simulink subsystem "DataSample"  (R2019b)
settings: Solver=VariableStepAuto  StartTime=0.0  StopTime=10.0  RelTol=1e-3
undefined symbols (not defined in the file or in its folder): __PRM__SERIALIZED__DATA__, SubsystemReferenceBlock
settings Model: Creator=VM  LastModifiedBy=VM

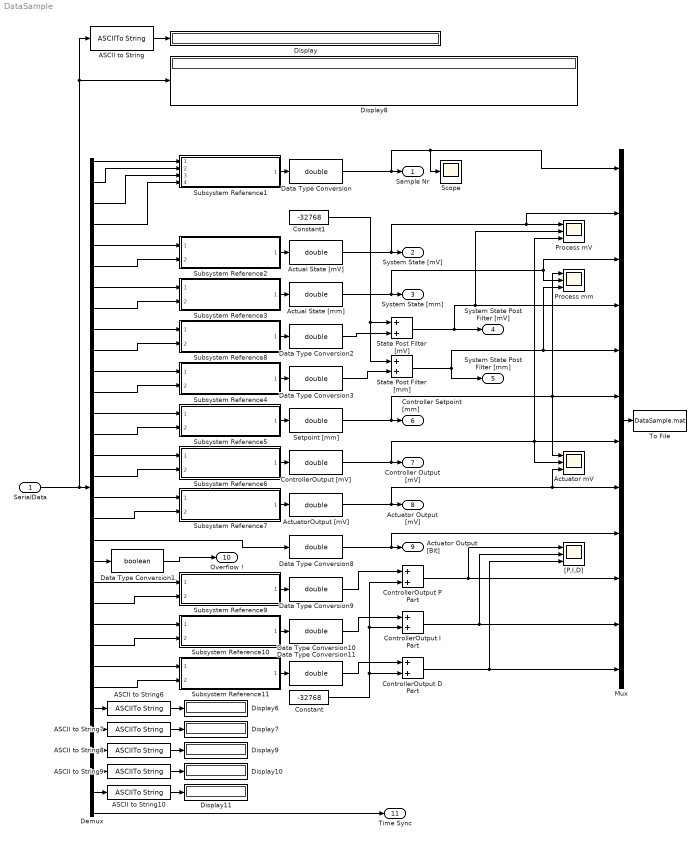
== system DataSample ==
  SerialData : Inport
  " Actual State [mV]" : DataTypeConversion  OutDataTypeStr=double
  " Actual State [mm]" : DataTypeConversion  OutDataTypeStr=double
  ASCII to String{,6..10} (6 alike) : ASCIIToString
  Actuator mV : Scope  NumInputPorts=3
  ActuatorOutput [mV] : DataTypeConversion  OutDataTypeStr=double
  Constant : Constant  Value=-32768
  Constant1 : Constant  Value=-32768
  ControllerOutput D Part : Sum
  ControllerOutput I Part : Sum
  ControllerOutput P Part : Sum
  ControllerOutput [mV] : DataTypeConversion  OutDataTypeStr=double
  Data Type Conversion{,2..3,8..11} (7 alike) : DataTypeConversion  OutDataTypeStr=double
  Data Type Conversion1 : DataTypeConversion  OutDataTypeStr=boolean
  Demux : Demux  Outputs=32
  Display{,6..11} (7 alike) : Display
      Display8 settings: Decimation=32
  Mux : Mux  Inputs=12
  Process mV : Scope  NumInputPorts=3
  Process mm : Scope  NumInputPorts=3
  Scope : Scope
  Setpoint [mm] : DataTypeConversion  OutDataTypeStr=double
  State Post Filter [mV] : Sum
  State Post Filter [mm] : Sum
  Subsystem Reference1 : Subsystem  BlockKeywords=__PRM__SERIALIZED__DATA__:SubsystemReferenceBlock  ReferencedSubsystem=DeserializeUINT32
  Subsystem Reference{2..11} (10 alike) : Subsystem  BlockKeywords=__PRM__SERIALIZED__DATA__:SubsystemReferenceBlock  ReferencedSubsystem=DeserializeUINT16
  To File : ToFile  Filename=DataSample.mat  MatrixName=DataSample  SaveFormat=Timeseries
  "[P,I,D]" : Scope  NumInputPorts=3
  Sample Nr : Outport
  System State [mV] : Outport  Port=2
  System State [mm] : Outport  Port=3
  System State Post Filter [mV] : Outport  Port=4
  System State Post Filter [mm] : Outport  Port=5
  Controller Setpoint [mm] : Outport  Port=6
  Controller Output [mV] : Outport  Port=7
  Actuator Output [mV] : Outport  Port=8
  Actuator Output [Bit] : Outport  Port=9
  Overflow ! : Outport  Port=10  OutDataTypeStr=boolean
  Time Sync : Outport  Port=11
  wires:
  SerialData/1 -> Demux/1, Display8/1, ASCII to String/1
  Demux/2 -> Subsystem Reference1/2
  Demux/1 -> Subsystem Reference1/1
  Demux/3 -> Subsystem Reference1/3
  Demux/4 -> Subsystem Reference1/4
  Demux/17 -> Subsystem Reference7/1
  Demux/18 -> Subsystem Reference7/2
  Subsystem Reference1/1 -> Data Type Conversion/1
  Subsystem Reference7/1 -> ActuatorOutput [mV]/1
  Demux/19 -> Data Type Conversion8/1
  Data Type Conversion/1 -> Sample Nr/1, Mux/1, Scope/1
  " Actual State [mV]"/1 -> System State [mV]/1, Process mV/1, Mux/2
  " Actual State [mm]"/1 -> System State [mm]/1, Mux/3, Process mm/2
  Setpoint [mm]/1 -> Controller Setpoint [mm]/1, Actuator mV/1, Mux/6, Process mm/1
  ControllerOutput [mV]/1 -> Controller Output [mV]/1, Process mV/3, Mux/7, Actuator mV/2
  ActuatorOutput [mV]/1 -> Actuator Output [mV]/1, Mux/8, Actuator mV/3
  Data Type Conversion8/1 -> Actuator Output [Bit]/1, Mux/9
  ASCII to String/1 -> Display/1
  Mux/1 -> To File/1
  Demux/32 -> Time Sync/1
  ASCII to String6/1 -> Display6/1
  Demux/27 -> ASCII to String6/1
  ASCII to String7/1 -> Display7/1
  Demux/28 -> ASCII to String7/1
  ASCII to String8/1 -> Display9/1
  Demux/29 -> ASCII to String8/1
  ASCII to String9/1 -> Display10/1
  Demux/30 -> ASCII to String9/1
  ASCII to String10/1 -> Display11/1
  Demux/31 -> ASCII to String10/1
  Subsystem Reference2/1 -> " Actual State [mV]"/1
  Subsystem Reference3/1 -> " Actual State [mm]"/1
  Subsystem Reference5/1 -> Setpoint [mm]/1
  Subsystem Reference6/1 -> ControllerOutput [mV]/1
  Demux/5 -> Subsystem Reference2/1
  Demux/6 -> Subsystem Reference2/2
  Demux/7 -> Subsystem Reference3/1
  Demux/9 -> Subsystem Reference8/1
  Demux/11 -> Subsystem Reference4/1
  Demux/13 -> Subsystem Reference5/1
  Demux/15 -> Subsystem Reference6/1
  Demux/16 -> Subsystem Reference6/2
  Demux/14 -> Subsystem Reference5/2
  Demux/12 -> Subsystem Reference4/2
  Demux/10 -> Subsystem Reference8/2
  Demux/8 -> Subsystem Reference3/2
  Demux/21 -> Subsystem Reference9/1
  Demux/22 -> Subsystem Reference9/2
  Demux/23 -> Subsystem Reference10/1
  Demux/24 -> Subsystem Reference10/2
  Demux/25 -> Subsystem Reference11/1
  Demux/26 -> Subsystem Reference11/2
  Subsystem Reference9/1 -> Data Type Conversion9/1
  Subsystem Reference10/1 -> Data Type Conversion10/1
  Subsystem Reference11/1 -> Data Type Conversion11/1
  Data Type Conversion9/1 -> ControllerOutput P Part/1
  Data Type Conversion11/1 -> ControllerOutput D Part/1
  Data Type Conversion10/1 -> ControllerOutput I Part/1
  Constant/1 -> ControllerOutput P Part/2, ControllerOutput I Part/2, ControllerOutput D Part/2
  ControllerOutput P Part/1 -> Mux/10, "[P,I,D]"/1
  ControllerOutput I Part/1 -> Mux/11, "[P,I,D]"/2
  ControllerOutput D Part/1 -> "[P,I,D]"/3, Mux/12
  Data Type Conversion1/1 -> Overflow !/1
  Demux/20 -> Data Type Conversion1/1
  State Post Filter [mV]/1 -> Process mV/2, Mux/4, System State Post Filter [mV]/1
  Constant1/1 -> State Post Filter [mm]/1, State Post Filter [mV]/1
  Subsystem Reference8/1 -> Data Type Conversion2/1
  Data Type Conversion2/1 -> State Post Filter [mV]/2
  Subsystem Reference4/1 -> Data Type Conversion3/1
  Data Type Conversion3/1 -> State Post Filter [mm]/2
  State Post Filter [mm]/1 -> System State Post Filter [mm]/1, Process mm/3, Mux/5
